simulink subsystem "Canard_Aerodynamics"  (R2025b)
settings: Solver=VariableStepAuto  StartTime=0.0  StopTime=10.0  RelTol=1e-3
values from neighbouring files (symbols this model uses):
  Fin_CoefficientsLookupTable = [ ... (first row only)    [data.m]
  Fin_CrossSectionArea = 0.0007    [data.m]
  Fin_OffsetFromCenter = 0.113    [data.m]
  Fin_SurfaceArea = 0.0050    (= 0.005)    [data.m]
  Fin_ZPos = -1.47    [data.m]
libraries: aerolibbdyn x1, vrlib x1
settings Model: Creator=Filip  LastModifiedBy=Filip

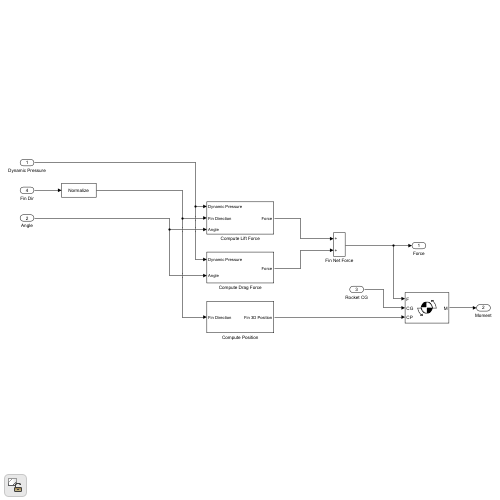
[thumbnail: Simulink's stored preview of the top-level diagram]
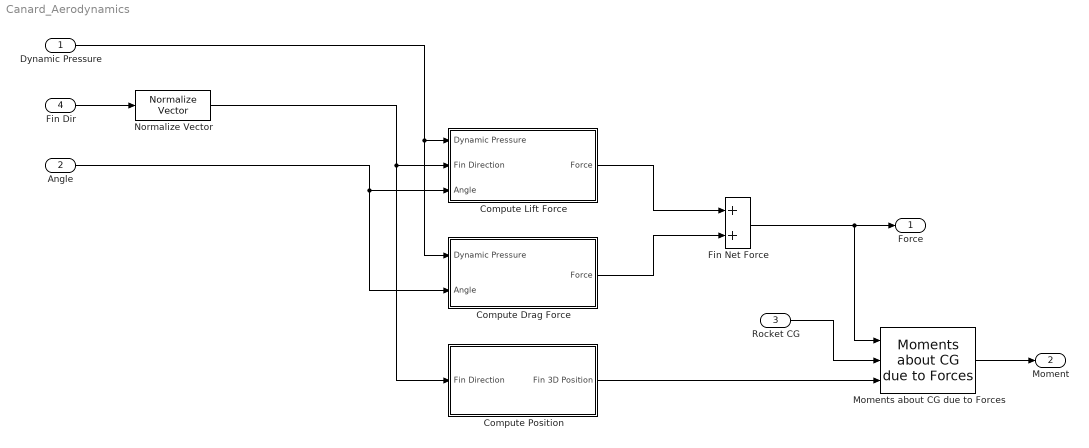
== system Canard_Aerodynamics ==
  Dynamic Pressure : Inport
  Angle : Inport  Port=2
  Rocket CG : Inport  Port=3
  Fin Dir : Inport  Port=4
  Compute Drag Force : Subsystem
  Compute Lift Force : Subsystem
  Compute Position : Subsystem
  Fin Net Force : Sum
  Moments about CG due to Forces : aerolibbdyn/Moments about CG  due to Forces
  Normalize Vector : vrlib/Utilities/Normalize Vector  maxzero=0
  Force : Outport
  Moment : Outport  Port=2
  wires:
  Moments about CG due to Forces/1 -> Moment/1
  Rocket CG/1 -> Moments about CG due to Forces/2
  Compute Position/1(Fin 3D Position) -> Moments about CG due to Forces/3
  Compute Lift Force/1(Force) -> Fin Net Force/1
  Compute Drag Force/1(Force) -> Fin Net Force/2
  Fin Net Force/1 -> Force/1, Moments about CG due to Forces/1
  Dynamic Pressure/1 -> Compute Lift Force/1(Dynamic Pressure), Compute Drag Force/1(Dynamic Pressure)
  Normalize Vector/1 -> Compute Lift Force/2(Fin Direction), Compute Position/1(Fin Direction)
  Fin Dir/1 -> Normalize Vector/1
  Angle/1 -> Compute Drag Force/2(Angle), Compute Lift Force/3(Angle)

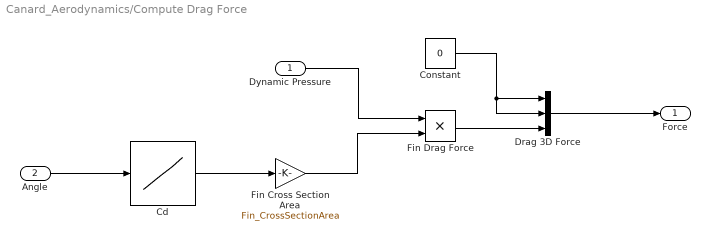
== system Canard_Aerodynamics/Compute Drag Force ==
  Dynamic Pressure : Inport
  Angle : Inport  Port=2
  Cd : Lookup_n-D  NumberOfTableDimensions=1  BreakpointsForDimension1=Fin_CoefficientsLookupTable(:, 1)  Table=Fin_CoefficientsLookupTable(:, 3)  ExtrapMethod=Clip  UseLastTableValue=on  InternalRulePriority=Speed  RndMeth=Simplest
  Constant : Constant  Value=0
  Drag 3D Force : Mux  Inputs=3
  Fin Cross Section Area : Gain  Gain=Fin_CrossSectionArea
  Fin Drag Force : Product
  Force : Outport
  wires:
  Angle/1 -> Cd/1
  Cd/1 -> Fin Cross Section Area/1
  Fin Cross Section Area/1 -> Fin Drag Force/2
  Dynamic Pressure/1 -> Fin Drag Force/1
  Constant/1 -> Drag 3D Force/1, Drag 3D Force/2
  Fin Drag Force/1 -> Drag 3D Force/3
  Drag 3D Force/1 -> Force/1

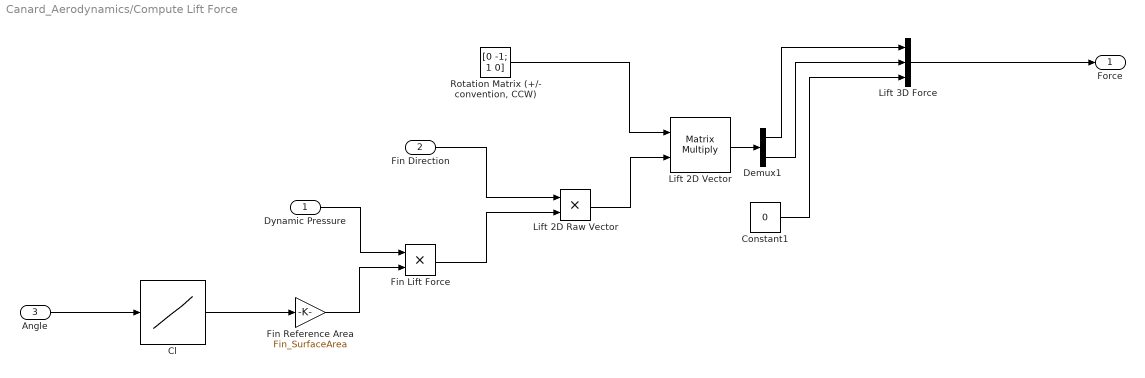
== system Canard_Aerodynamics/Compute Lift Force ==
  Dynamic Pressure : Inport
  Fin Direction : Inport  Port=2
  Angle : Inport  Port=3
  Cl : Lookup_n-D  NumberOfTableDimensions=1  BreakpointsForDimension1=Fin_CoefficientsLookupTable(:, 1)  Table=Fin_CoefficientsLookupTable(:, 2)  ExtrapMethod=Clip  UseLastTableValue=on  InternalRulePriority=Speed  RndMeth=Simplest
  Constant1 : Constant  Value=0
  Demux1 : Demux  Outputs=2
  Fin Lift Force : Product
  Fin Reference Area : Gain  Gain=Fin_SurfaceArea
  Lift 2D Raw Vector : Product
  Lift 2D Vector : Product  Multiplication=Matrix(*)
  Lift 3D Force : Mux  Inputs=3
  "Rotation Matrix (+/- convention, CCW)" : Constant  Value=[0 -1; 1 0]
  Force : Outport
  wires:
  Angle/1 -> Cl/1
  Cl/1 -> Fin Reference Area/1
  Fin Reference Area/1 -> Fin Lift Force/2
  Fin Direction/1 -> Lift 2D Raw Vector/1
  Dynamic Pressure/1 -> Fin Lift Force/1
  Demux1/1 -> Lift 3D Force/1
  Lift 2D Vector/1 -> Demux1/1
  Constant1/1 -> Lift 3D Force/3
  Lift 2D Raw Vector/1 -> Lift 2D Vector/2
  Fin Lift Force/1 -> Lift 2D Raw Vector/2
  Lift 3D Force/1 -> Force/1
  Demux1/2 -> Lift 3D Force/2
  "Rotation Matrix (+/- convention, CCW)"/1 -> Lift 2D Vector/1

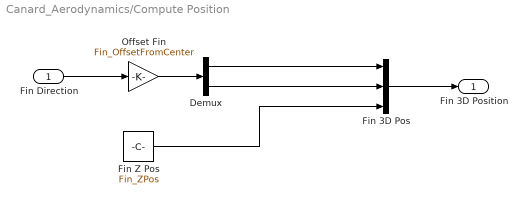
== system Canard_Aerodynamics/Compute Position ==
  Fin Direction : Inport
  Demux : Demux  Outputs=2
  Fin 3D Pos : Mux  Inputs=3
  Fin Z Pos : Constant  Value=Fin_ZPos
  Offset Fin : Gain  Gain=Fin_OffsetFromCenter
  Fin 3D Position : Outport
  wires:
  Fin 3D Pos/1 -> Fin 3D Position/1
  Fin Direction/1 -> Offset Fin/1
  Demux/1 -> Fin 3D Pos/1
  Demux/2 -> Fin 3D Pos/2
  Fin Z Pos/1 -> Fin 3D Pos/3
  Offset Fin/1 -> Demux/1
